simulink model "myPID"  (R2014a)
settings: Solver=ode45  StartTime=0.0  StopTime=10.0  RelTol=1e-3
settings Model: Creator=Administrator  LastModifiedBy=Administrator

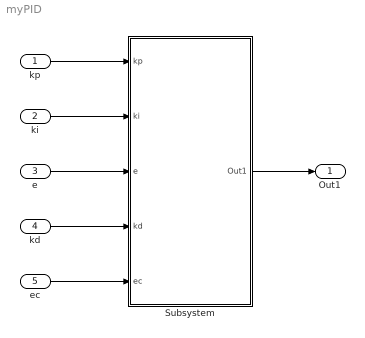
== system myPID ==
  kp : Inport
  ki : Inport  Port=2
  e : Inport  Port=3
  kd : Inport  Port=4
  ec : Inport  Port=5
  Subsystem : Subsystem
  Out1 : Outport
  wires:
  kp/1 -> Subsystem/1(kp)
  ki/1 -> Subsystem/2(ki)
  e/1 -> Subsystem/3(e)
  kd/1 -> Subsystem/4(kd)
  ec/1 -> Subsystem/5(ec)
  Subsystem/1(Out1) -> Out1/1

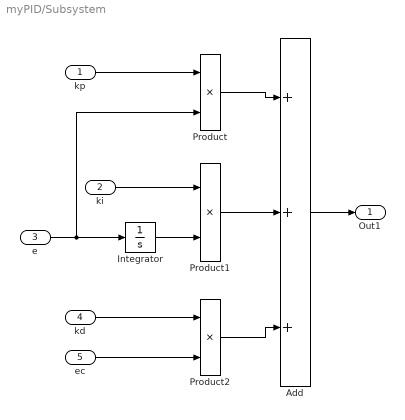
== system myPID/Subsystem ==
  kp : Inport
  ki : Inport  Port=2
  e : Inport  Port=3
  kd : Inport  Port=4
  ec : Inport  Port=5
  Add : Sum  Inputs=+++
  Integrator : Integrator
  Product : Product
  Product1 : Product
  Product2 : Product
  Out1 : Outport
  wires:
  kd/1 -> Product2/1
  Integrator/1 -> Product1/2
  e/1 -> Product/2, Integrator/1
  ec/1 -> Product2/2
  Product/1 -> Add/1
  Product1/1 -> Add/2
  Product2/1 -> Add/3
  Add/1 -> Out1/1
  ki/1 -> Product1/1
  kp/1 -> Product/1
